simulink model "ProSpec2dla"  (R2016a)
settings: Solver=ode23  SolverMode=SingleTasking  StartTime=0.0  StopTime=1000  RelTol=1e-5
undefined symbols (not defined in the file): K1, R
libraries: simulink x1
settings Model: Creator=kajaczekmackbookpro  LastModifiedBy=kajaczekmackbookpro
settings DebuggingCC: SFUnexpectedBacktrackingDiag=error  SFNoUnconditionalDefaultTransitionDiag=error
settings SFSimCC: SimUseLocalCustomCode=on
settings RTWCC: RTWUseLocalCustomCode=on
settings GRTTargetCC: TargetLangStandard=C99 (ISO)  GeneratePreprocessorConditionals=Use local settings
settings ConfigComp: CovMetricSettings=dwe  CovHtmlReporting=off  CovSaveCumulativeToWorkspaceVar=off  CovSaveSingleToWorkspaceVar=off  CovExternalEMLEnable=on

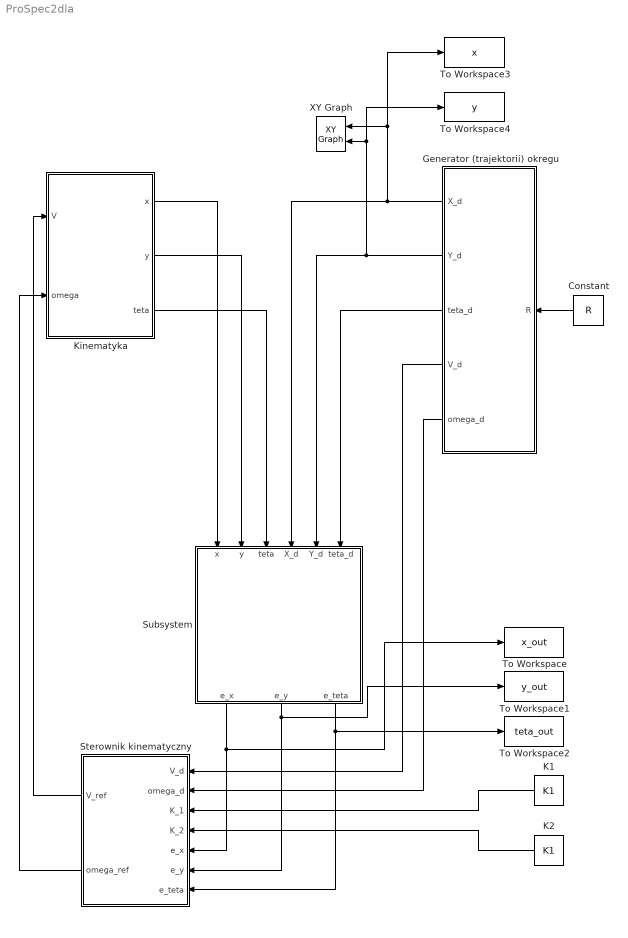
== system ProSpec2dla ==
  Constant : Constant  Value=R
  Generator (trajektorii) okregu : Subsystem
  K1 : Constant  Value=K1
  K2 : Constant  Value=K1
  Kinematyka : Subsystem
  Sterownik kinematyczny : Subsystem
  Subsystem : Subsystem
  To Workspace : ToWorkspace  VariableName=x_out  SaveFormat=Timeseries  SampleTime=-1
  To Workspace1 : ToWorkspace  VariableName=y_out  SaveFormat=Timeseries  SampleTime=-1
  To Workspace2 : ToWorkspace  VariableName=teta_out  SaveFormat=Timeseries  SampleTime=-1
  To Workspace3 : ToWorkspace  VariableName=x  SaveFormat=Timeseries  SampleTime=-1
  To Workspace4 : ToWorkspace  VariableName=y  SaveFormat=Timeseries  SampleTime=-1
  XY Graph : simulink/Sinks/XY Graph  xmin=-6  xmax=6  ymin=-6  ymax=6  st=-1
  wires:
  Constant/1 -> Generator (trajektorii) okregu/1(R)
  Generator (trajektorii) okregu/1(X_d) -> Subsystem/4(X_d), To Workspace3/1, XY Graph/1
  Generator (trajektorii) okregu/2(Y_d) -> Subsystem/5(Y_d), To Workspace4/1, XY Graph/2
  Kinematyka/1(x) -> Subsystem/1(x)
  Kinematyka/2(y) -> Subsystem/2(y)
  Kinematyka/3(teta) -> Subsystem/3(teta)
  Generator (trajektorii) okregu/3(teta_d) -> Subsystem/6(teta_d)
  Sterownik kinematyczny/1(V_ref) -> Kinematyka/1(V)
  Sterownik kinematyczny/2(omega_ref) -> Kinematyka/2(omega)
  Generator (trajektorii) okregu/4(V_d) -> Sterownik kinematyczny/1(V_d)
  Generator (trajektorii) okregu/5(omega_d) -> Sterownik kinematyczny/2(omega_d)
  Subsystem/1(e_x) -> To Workspace/1, Sterownik kinematyczny/5(e_x)
  Subsystem/2(e_y) -> Sterownik kinematyczny/6(e_y), To Workspace1/1
  Subsystem/3(e_teta) -> To Workspace2/1, Sterownik kinematyczny/7(e_teta)
  K1/1 -> Sterownik kinematyczny/3(K_1)
  K2/1 -> Sterownik kinematyczny/4(K_2)

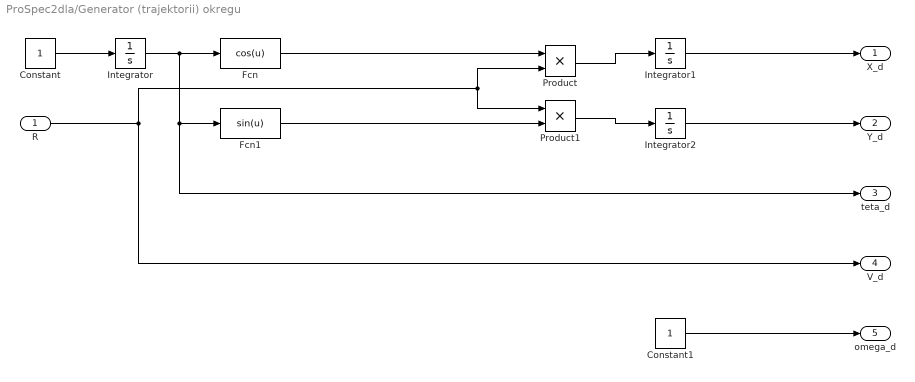
== system ProSpec2dla/Generator (trajektorii) okregu ==
  R : Inport
  Constant : Constant
  Constant1 : Constant
  Fcn : Fcn  Expr=cos(u)
  Fcn1 : Fcn  Expr=sin(u)
  Integrator : Integrator
  Integrator1 : Integrator
  Integrator2 : Integrator  InitialCondition=-R
  Product : Product
  Product1 : Product
  X_d : Outport
  Y_d : Outport  Port=2
  teta_d : Outport  Port=3
  V_d : Outport  Port=4
  omega_d : Outport  Port=5
  wires:
  Constant/1 -> Integrator/1
  Product1/1 -> Integrator2/1
  Integrator2/1 -> Y_d/1
  Fcn/1 -> Product/1
  Product/1 -> Integrator1/1
  Constant1/1 -> omega_d/1
  Integrator1/1 -> X_d/1
  Fcn1/1 -> Product1/2
  Integrator/1 -> teta_d/1, Fcn1/1, Fcn/1
  R/1 -> V_d/1, Product1/1, Product/2

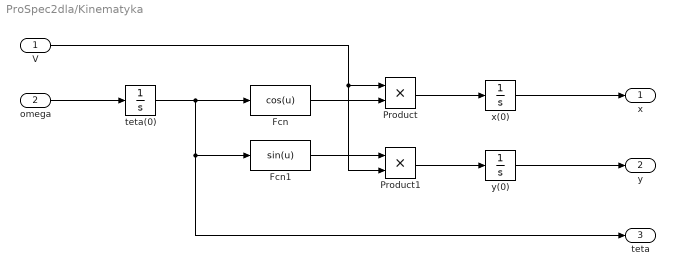
== system ProSpec2dla/Kinematyka ==
  V : Inport
  omega : Inport  Port=2
  Fcn : Fcn  Expr=cos(u)
  Fcn1 : Fcn  Expr=sin(u)
  Product : Product
  Product1 : Product
  teta(0) : Integrator
  x(0) : Integrator
  y(0) : Integrator  InitialCondition=-R
  x : Outport
  y : Outport  Port=2
  teta : Outport  Port=3
  wires:
  Fcn/1 -> Product/2
  Product/1 -> x(0)/1
  Fcn1/1 -> Product1/1
  teta(0)/1 -> teta/1, Fcn1/1, Fcn/1
  V/1 -> Product1/2, Product/1
  y(0)/1 -> y/1
  omega/1 -> teta(0)/1
  x(0)/1 -> x/1
  Product1/1 -> y(0)/1

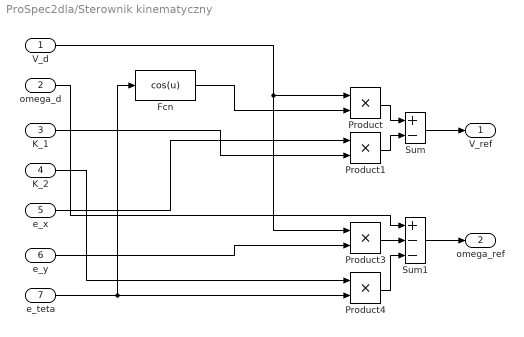
== system ProSpec2dla/Sterownik kinematyczny ==
  V_d : Inport
  omega_d : Inport  Port=2
  K_1 : Inport  Port=3
  K_2 : Inport  Port=4
  e_x : Inport  Port=5
  e_y : Inport  Port=6
  e_teta : Inport  Port=7
  Fcn : Fcn  Expr=cos(u)
  Product{,1,3..4} (4 alike) : Product
  Sum : Sum  Inputs=+-
  Sum1 : Sum  Inputs=+--
  V_ref : Outport
  omega_ref : Outport  Port=2
  wires:
  Sum1/1 -> omega_ref/1
  K_1/1 -> Product1/2
  Product1/1 -> Sum/2
  e_y/1 -> Product3/2
  e_teta/1 -> Product4/2, Fcn/1
  omega_d/1 -> Sum1/1
  Product3/1 -> Sum1/2
  Fcn/1 -> Product/2
  V_d/1 -> Product3/1, Product/1
  Sum/1 -> V_ref/1
  K_2/1 -> Product4/1
  Product/1 -> Sum/1
  Product4/1 -> Sum1/3
  e_x/1 -> Product1/1

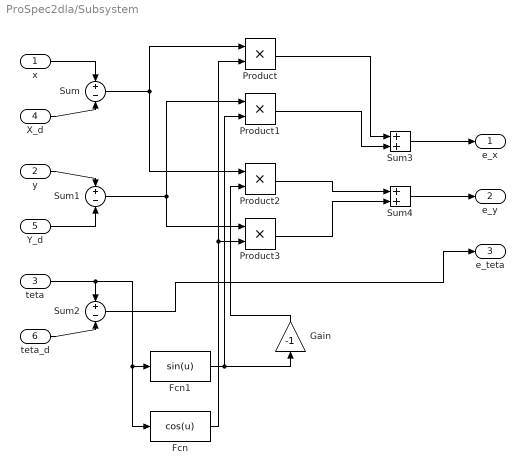
== system ProSpec2dla/Subsystem ==
  x : Inport
  y : Inport  Port=2
  teta : Inport  Port=3
  X_d : Inport  Port=4
  Y_d : Inport  Port=5
  teta_d : Inport  Port=6
  Fcn : Fcn  Expr=cos(u)
  Fcn1 : Fcn  Expr=sin(u)
  Gain : Gain  Gain=-1
  Product{,1..3} (4 alike) : Product
  Sum : Sum  Inputs=+-
  Sum1 : Sum  Inputs=+-
  Sum2 : Sum  Inputs=+-
  Sum3 : Sum
  Sum4 : Sum
  e_x : Outport
  e_y : Outport  Port=2
  e_teta : Outport  Port=3
  wires:
  X_d/1 -> Sum/2
  Y_d/1 -> Sum1/2
  Product3/1 -> Sum4/2
  teta_d/1 -> Sum2/2
  Product1/1 -> Sum3/2
  Fcn1/1 -> Gain/1, Product1/2
  Sum1/1 -> Product3/1, Product1/1
  Sum/1 -> Product/1, Product2/1
  teta/1 -> Fcn/1, Fcn1/1, Sum2/1
  Sum4/1 -> e_y/1
  Product2/1 -> Sum4/1
  x/1 -> Sum/1
  Sum2/1 -> e_teta/1
  Fcn/1 -> Product3/2, Product/2
  Gain/1 -> Product2/2
  Product/1 -> Sum3/1
  y/1 -> Sum1/1
  Sum3/1 -> e_x/1
